simulink model "closed-loop_mechan_ventilator"  (R2018b)
settings: Solver=VariableStepAuto  StartTime=0.0  StopTime=10.0  RelTol=1e-3  EnableMultiTasking=on
libraries: cstblocks x9, dsparch4 x2, simulink x1
settings Model: Creator=bhajdarevic  LastModifiedBy=bhajd
settings DataIOCC: SaveFormat=Array
settings OptimizationCC: LifeSpan=inf
settings DebuggingCC: SFUnexpectedBacktrackingDiag=warning  SFNoUnconditionalDefaultTransitionDiag=warning  SFExecutionAtInitializationDiag=none
settings SFSimCC: SimUseLocalCustomCode=off
settings RTWCC: RTWUseLocalCustomCode=off
settings CodeAppCC: StateflowObjectComments=on
settings GRTTargetCC: TargetLangStandard=C89/C90 (ANSI)  GeneratePreprocessorConditionals=Disable all
settings ConfigComp: CovMetricSettings=dw  CovHtmlReporting=on  CovSaveCumulativeToWorkspaceVar=on  CovSaveSingleToWorkspaceVar=on  CovExternalEMLEnable=off

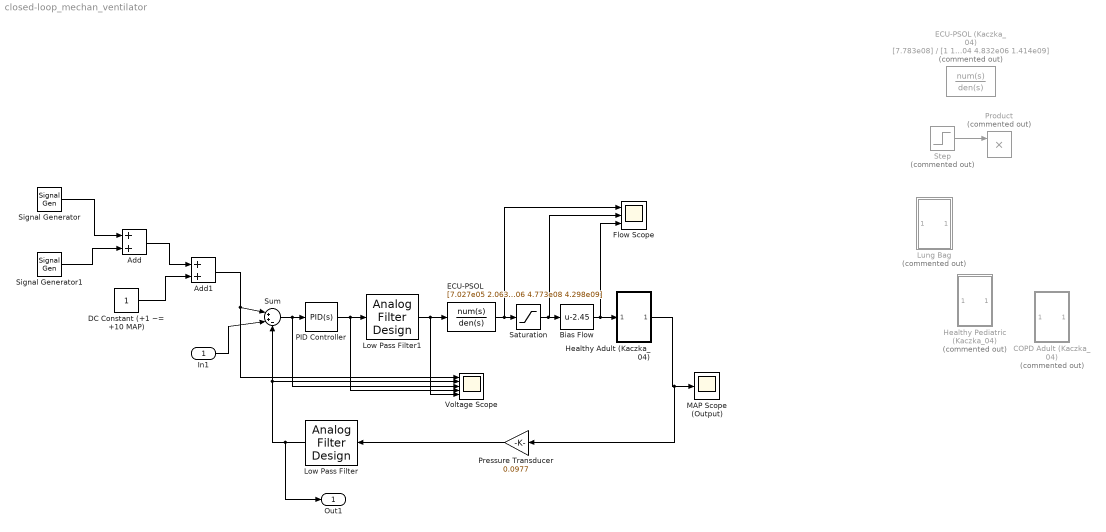
== system closed-loop_mechan_ventilator ==
  In1 : Inport
  Add : Sum
  Add1 : Sum
  Bias Flow : Bias  Bias=-2.45
  COPD Adult (Kaczka_04) : Subsystem  Commented=on
  DC Constant (+1 ~= +10 MAP) : Constant
  ECU-PSOL : TransferFcn  Numerator=[7.027e05 2.063e08 2.763e09]  Denominator=[1 270.6 8.645e04 7.733e06 4.773e08 4.298e09]
  ECU-PSOL (Kaczka_04) : TransferFcn  Commented=on  Numerator=[7.783e08]  Denominator=[1 160.1 9.043e04 4.832e06 1.414e09]
  Flow Scope : Scope  NumInputPorts=3
  Healthy Adult (Kaczka_04) : Subsystem
  Healthy Pediatric (Kaczka_04) : Subsystem  Commented=on
  Low Pass Filter : dsparch4/Analog Filter Design  method=Butterworth  filttype=Lowpass  N=8  Wlo=314  Whi=80  Rp=2  Rs=40
  Low Pass Filter1 : dsparch4/Analog Filter Design  method=Butterworth  filttype=Lowpass  N=8  Wlo=314  Whi=80  Rp=2  Rs=40
  Lung Bag : Subsystem  Commented=on
  MAP Scope (Output) : Scope
  PID Controller : simulink/Continuous/PID Controller  Controller=PID  Form=Parallel  TimeDomain=Continuous-time  SampleTime=-1  IntegratorMethod=Forward Euler  FilterMethod=Forward Euler  ControllerParametersSource=internal  P=1.04  I=4.81  D=0  UseFilter=on  N=1  TunerSelectOption=Transfer Function Based (PID Tuner App)  InitialConditionSource=internal  InitialConditionForIntegrator=0  InitialConditionForFilter=0  DifferentiatorICPrevScaledInput=0  ExternalReset=none  TrackingMode=off  Kt=1  LimitOutput=off  UpperSaturationLimit=inf  LowerSaturationLimit=-inf  LinearizeAsGain=on  AntiWindupMode=none  Kb=1  POutMin=[]  POutMax=[]  IOutMin=[]  IOutMax=[]  DOutMin=[]  DOutMax=[]  NOutMin=[]  NOutMax=[]  SumOutMin=[]  SumOutMax=[]  SaturationOutMin=[]  SaturationOutMax=[]  PParamMin=[]  PParamMax=[]  IParamMin=[]  IParamMax=[]  DParamMin=[]  DParamMax=[]  NParamMin=[]  NParamMax=[]  KbParamMin=[]  KbParamMax=[]  KtParamMin=[]  KtParamMax=[]  KbOutMin=[]  KbOutMax=[]  KtOutMin=[]  KtOutMax=[]  IntegratorOutMin=[]  IntegratorOutMax=[]  FilterOutMin=[]  FilterOutMax=[]  SumI1OutMin=[]  SumI1OutMax=[]  SumI2OutMin=[]  SumI2OutMax=[]  SumI3OutMin=[]  SumI3OutMax=[]  SumI4OutMin=[]  SumI4OutMax=[]  SumDOutMin=[]  SumDOutMax=[]  DifferentiatorOutMin=[]  DifferentiatorOutMax=[]  FilterDiffOutCoefMin=[]  FilterDiffOutCoefMax=[]  ReciprocalOutMin=[]  ReciprocalOutMax=[]  SumDenOutMin=[]  SumDenOutMax=[]  SumNumOutMin=[]  SumNumOutMax=[]  DivideOutMin=[]  DivideOutMax=[]  IntegratorContinuousStateAttributes=''  IntegratorStateMustResolveToSignalObject=off  IntegratorRTWStateStorageClass=Auto  FilterContinuousStateAttributes=''  FilterStateMustResolveToSignalObject=off  FilterRTWStateStorageClass=Auto  ParallelPVariant=InternalParameters  IdealPVariant=Disabled  IVariant=InternalParameters  DVariant=InternalParameters  IntegratorVariant=Continuous  SatVariant=Disabled  AWVariant=Passthrough  PCopyVariant=Disabled  TRVariant=Disabled  FdbkBlocksVariant=Forward  IdealPFdbkVariant=Disabled  SatFdbkVariant=Disabled  DerivativeFilterVariant=ContFilter  NVariant=InternalParameters  NCopyVariant=Disabled  FilterICVariant=InternalICsFilter  IntegratorICVariant=InternalICs  ExternalResetVariant=Disabled  TRSumVariant=Passthrough  SumFdbkVariant=Disabled  SumVariant=Sum_PID
  Pressure Transducer : Gain  Gain=0.0977
  Product : Product  Commented=on
  Saturation : Saturate  UpperLimit=4.7  LowerLimit=0
  Signal Generator : SignalGenerator  Amplitude=0.25  Frequency=2  Units=rad/sec
  Signal Generator1 : SignalGenerator  Amplitude=0  Units=rad/sec
  Step : Step  Commented=on  Time=10  SampleTime=0
  Sum : Sum  Inputs=|++-
  Voltage Scope : Scope  NumInputPorts=5
  Out1 : Outport
  wires:
  Signal Generator/1 -> Add/1
  Signal Generator1/1 -> Add/2
  Add/1 -> Add1/1
  DC Constant (+1 ~= +10 MAP)/1 -> Add1/2
  Add1/1 -> Sum/1, Voltage Scope/1
  Pressure Transducer/1 -> Low Pass Filter/1
  Low Pass Filter/1 -> Out1/1, Sum/3, Voltage Scope/2
  In1/1 -> Sum/2
  Saturation/1 -> Flow Scope/2, Bias Flow/1
  Step/1 -> Product/1
  Bias Flow/1 -> Healthy Adult (Kaczka_04)/1(In1), Flow Scope/3
  Sum/1 -> PID Controller/1, Voltage Scope/3
  PID Controller/1 -> Voltage Scope/4, Low Pass Filter1/1
  ECU-PSOL/1 -> Flow Scope/1, Saturation/1
  Healthy Adult (Kaczka_04)/1(Out1) -> Pressure Transducer/1, MAP Scope (Output)/1
  Low Pass Filter1/1 -> Voltage Scope/5, ECU-PSOL/1

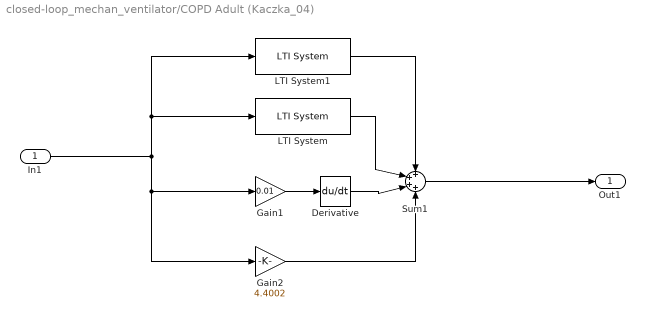
== system closed-loop_mechan_ventilator/COPD Adult (Kaczka_04) ==
  In1 : Inport
  Derivative : Derivative
  Gain1 : Gain  Gain=0.01
  Gain2 : Gain  Gain=4.4002
  LTI System : cstblocks/LTI System  sys=tf(691.2,[1 26.98])  IC=[]
  LTI System1 : cstblocks/LTI System  sys=tf(30.02,[1 0])  IC=[]
  Sum1 : Sum  Inputs=++++
  Out1 : Outport
  wires:
  LTI System/1 -> Sum1/2
  Gain2/1 -> Sum1/4
  Derivative/1 -> Sum1/3
  LTI System1/1 -> Sum1/1
  In1/1 -> Gain1/1, Gain2/1, LTI System/1, LTI System1/1
  Sum1/1 -> Out1/1
  Gain1/1 -> Derivative/1

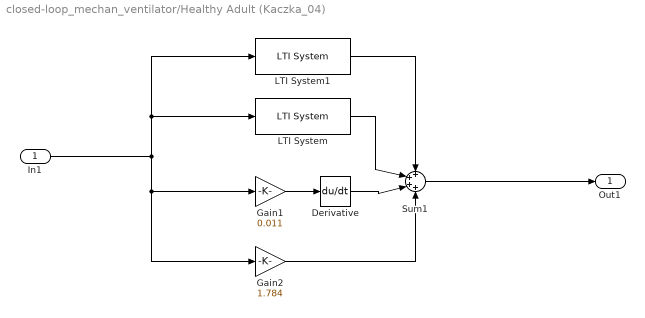
== system closed-loop_mechan_ventilator/Healthy Adult (Kaczka_04) ==
  In1 : Inport
  Derivative : Derivative
  Gain1 : Gain  Gain=0.011
  Gain2 : Gain  Gain=1.784
  LTI System : cstblocks/LTI System  sys=tf(17.5,[1 3.27])  IC=[]
  LTI System1 : cstblocks/LTI System  sys=tf(31.25,[1 0])  IC=[]
  Sum1 : Sum  Inputs=++++
  Out1 : Outport
  wires:
  LTI System/1 -> Sum1/2
  Gain2/1 -> Sum1/4
  Derivative/1 -> Sum1/3
  LTI System1/1 -> Sum1/1
  In1/1 -> Gain1/1, Gain2/1, LTI System/1, LTI System1/1
  Sum1/1 -> Out1/1
  Gain1/1 -> Derivative/1

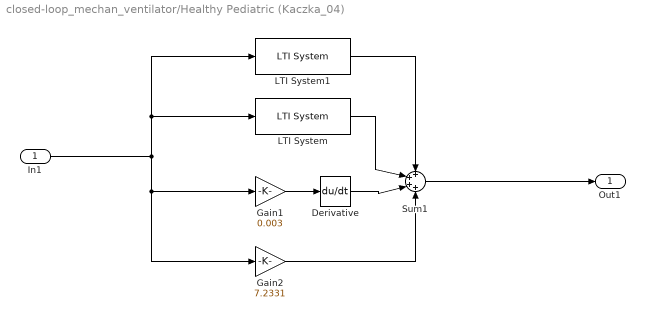
== system closed-loop_mechan_ventilator/Healthy Pediatric (Kaczka_04) ==
  In1 : Inport
  Derivative : Derivative
  Gain1 : Gain  Gain=0.003
  Gain2 : Gain  Gain=7.2331
  LTI System : cstblocks/LTI System  sys=tf(57.63,[1 2.31])  IC=[]
  LTI System1 : cstblocks/LTI System  sys=tf(122.1,[1 0])  IC=[]
  Sum1 : Sum  Inputs=++++
  Out1 : Outport
  wires:
  LTI System/1 -> Sum1/2
  Gain2/1 -> Sum1/4
  Derivative/1 -> Sum1/3
  LTI System1/1 -> Sum1/1
  In1/1 -> Gain1/1, Gain2/1, LTI System/1, LTI System1/1
  Sum1/1 -> Out1/1
  Gain1/1 -> Derivative/1

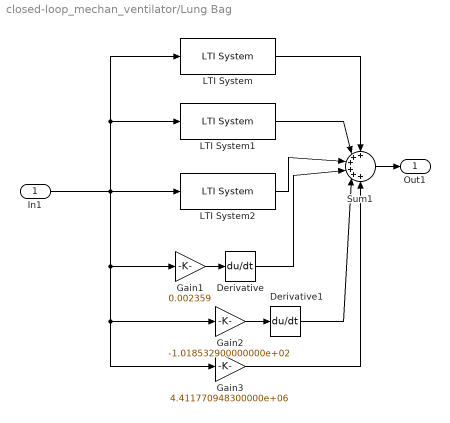
== system closed-loop_mechan_ventilator/Lung Bag ==
  In1 : Inport
  Derivative : Derivative
  Derivative1 : Derivative
  Gain1 : Gain  Gain=0.002359
  Gain2 : Gain  Gain=-1.018532900000000e+02
  Gain3 : Gain  Gain=4.411770948300000e+06
  LTI System : cstblocks/LTI System  sys=tf(-1.910612726658902e+11,[1 -(-4.330717368252098e+04)])  IC=[]
  LTI System1 : cstblocks/LTI System  sys=tf(4.996431515273606,[1 -(-2.761848467008354)])  IC=[]
  LTI System2 : cstblocks/LTI System  sys=tf(44.526474518135387,[1 -(-0.064469012023054)])  IC=[]
  Sum1 : Sum  Inputs=++++++
  Out1 : Outport
  wires:
  LTI System2/1 -> Sum1/3
  LTI System/1 -> Sum1/1
  LTI System1/1 -> Sum1/2
  Gain1/1 -> Derivative/1
  Gain3/1 -> Sum1/6
  In1/1 -> Gain2/1, Gain3/1, Gain1/1, LTI System2/1, LTI System1/1, LTI System/1
  Sum1/1 -> Out1/1
  Derivative/1 -> Sum1/4
  Gain2/1 -> Derivative1/1
  Derivative1/1 -> Sum1/5
